simulink model "IMU"  (R2019b)
settings: Solver=VariableStepAuto  StartTime=0.0  StopTime=10.0  RelTol=1e-3
settings Model: Creator=guy-m  LastModifiedBy=guy-m

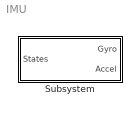
== system IMU ==
  Subsystem : Subsystem

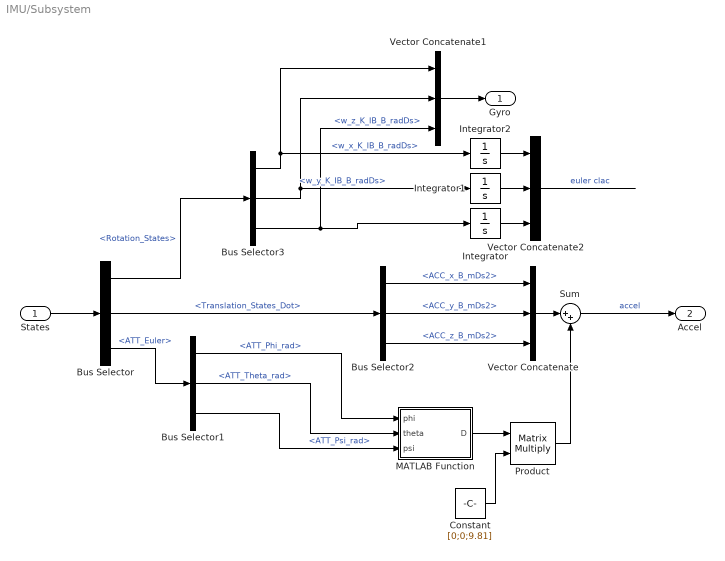
== system IMU/Subsystem ==
  States : Inport
  Bus Selector : BusSelector  OutputSignals=Rigid_Body_States.Rotation_States,Rigid_Body_States.Translation_States_Dot,Rigid_Body_States.Attitude_States.ATT_Euler
  Bus Selector1 : BusSelector  OutputSignals=ATT_Phi_rad,ATT_Theta_rad,ATT_Psi_rad
  Bus Selector2 : BusSelector  OutputSignals=ACC_x_B_mDs2,ACC_y_B_mDs2,ACC_z_B_mDs2
  Bus Selector3 : BusSelector  OutputSignals=w_x_K_IB_B_radDs,w_y_K_IB_B_radDs,w_z_K_IB_B_radDs
  Constant : Constant  Value=[0;0;9.81]
  Integrator : Integrator
  Integrator1 : Integrator  InitialCondition=1.356
  Integrator2 : Integrator
  MATLAB Function : MATLAB Function  TreatAsAtomicUnit=on
  Product : Product  Multiplication=Matrix(*)
  Sum : Sum  Inputs=|++
  Vector Concatenate : Concatenate  NumInputs=3
  Vector Concatenate1 : Concatenate  NumInputs=3
  Vector Concatenate2 : Concatenate  NumInputs=3
  Gyro : Outport
  Accel : Outport  Port=2
  wires:
  States/1 -> Bus Selector/1
  Bus Selector/2 -> Bus Selector2/1  "<Translation_States_Dot>"
  Bus Selector/3 -> Bus Selector1/1  "<ATT_Euler>"
  Bus Selector1/1 -> MATLAB Function/1(phi)  "<ATT_Phi_rad>"
  Bus Selector1/2 -> MATLAB Function/2(theta)  "<ATT_Theta_rad>"
  Bus Selector1/3 -> MATLAB Function/3(psi)  "<ATT_Psi_rad>"
  Constant/1 -> Product/2
  MATLAB Function/1(D) -> Product/1
  Product/1 -> Sum/2
  Bus Selector2/1 -> Vector Concatenate/1  "<ACC_x_B_mDs2>"
  Bus Selector2/2 -> Vector Concatenate/2  "<ACC_y_B_mDs2>"
  Bus Selector2/3 -> Vector Concatenate/3  "<ACC_z_B_mDs2>"
  Vector Concatenate/1 -> Sum/1
  Sum/1 -> Accel/1  "accel"
  Bus Selector/1 -> Bus Selector3/1  "<Rotation_States>"
  Bus Selector3/1 -> Integrator2/1, Vector Concatenate1/1  "<w_x_K_IB_B_radDs>"
  Bus Selector3/2 -> Integrator1/1, Vector Concatenate1/2  "<w_y_K_IB_B_radDs>"
  Bus Selector3/3 -> Integrator/1, Vector Concatenate1/3  "<w_z_K_IB_B_radDs>"
  Vector Concatenate1/1 -> Gyro/1
  Integrator2/1 -> Vector Concatenate2/1
  Integrator1/1 -> Vector Concatenate2/2
  Integrator/1 -> Vector Concatenate2/3
  Vector Concatenate2/1 -> ?  "euler clac"

== matlab function IMU/Subsystem/MATLAB Function ==
  data: phi input; theta input; D output; psi input
function D = fcn(phi, theta, psi)

D1 = [cos(theta)*cos(psi) cos(theta)*sin(psi) -sin(theta)];
D2 = [sin(phi)*sin(theta)*cos(psi)-cos(phi)*sin(psi) sin(phi)*sin(theta)*sin(psi)+cos(phi)*cos(psi) sin(phi)*cos(theta)];
D3 = [cos(phi)*sin(theta)*cos(psi)+sin(phi)*sin(psi) cos(phi)*sin(theta)*sin(psi)-sin(phi)*cos(psi) cos(phi)*cos(theta)];
D = [D1;D2;D3];
